simulink model "NonLin1C"  (R2019b)
settings: Solver=ode15s  StartTime=0.0  StopTime=200  FixedStep=0.1  RelTol=1e-3
values from neighbouring files (symbols this model uses):
  A_n = 0.05 * pi / 180    (= 0.000872664625997)    [Proj1C.m]
  g = 9.81    [Proj1C.m]
  K = 3    [Proj1C.m]
  L = 1    [Proj1C.m]
  M = 0.06    [Proj1C.m]
  omega_n = 200    [Proj1C.m]
  w_nonlin = W/8    (= 0.0109)    [Proj1C.m]
libraries: cstblocks x1
settings Model: NumberOfSteps=10  Creator=kmfrick  LastModifiedBy=kmfrick
settings SolverCC: ConcurrentTasks=on

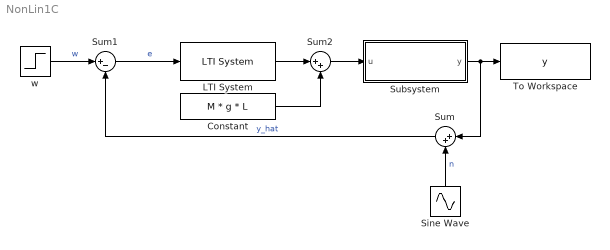
== system NonLin1C ==
  Constant : Constant  Value=M * g * L
  LTI System : cstblocks/LTI System  sys=R_opt  IC=[]
  Sine Wave : Sin  Amplitude=A_n  Frequency=omega_n  SampleTime=0
  Subsystem : Subsystem
  Sum : Sum  Inputs=|++
  Sum1 : Sum  Inputs=|+-
  Sum2 : Sum  Inputs=|++
  To Workspace : ToWorkspace  VariableName=y  SaveFormat=Timeseries  SampleTime=-1
  w : Step  Time=2  Before=pi/2  After=w_nonlin + pi/2  SampleTime=0
  wires:
  Sine Wave/1 -> Sum/2  "n"
  Sum/1 -> Sum1/2  "y_hat"
  Sum1/1 -> LTI System/1  "e"
  LTI System/1 -> Sum2/1
  Constant/1 -> Sum2/2
  w/1 -> Sum1/1  "w"
  Sum2/1 -> Subsystem/1(u)
  Subsystem/1(y) -> To Workspace/1, Sum/1

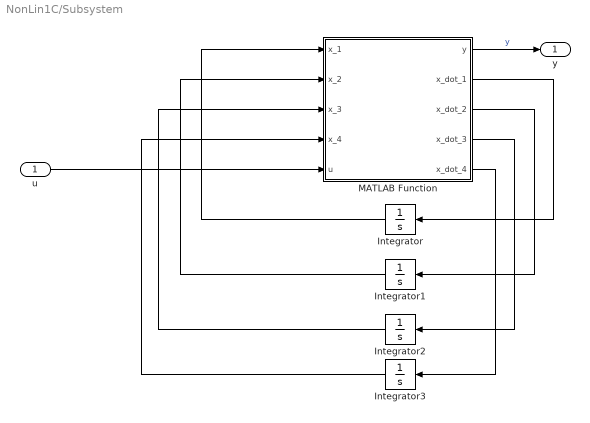
== system NonLin1C/Subsystem ==
  u : Inport
  Integrator : Integrator  InitialCondition=pi/2
  Integrator1 : Integrator
  Integrator2 : Integrator  InitialCondition=M *g * L / K + pi/2
  Integrator3 : Integrator
  MATLAB Function : MATLAB Function  TreatAsAtomicUnit=on
  y : Outport
  wires:
  Integrator1/1 -> MATLAB Function/2(x_2)
  MATLAB Function/3(x_dot_2) -> Integrator1/1
  MATLAB Function/5(x_dot_4) -> Integrator3/1
  Integrator/1 -> MATLAB Function/1(x_1)
  MATLAB Function/4(x_dot_3) -> Integrator2/1
  Integrator2/1 -> MATLAB Function/3(x_3)
  MATLAB Function/2(x_dot_1) -> Integrator/1
  Integrator3/1 -> MATLAB Function/4(x_4)
  u/1 -> MATLAB Function/5(u)
  MATLAB Function/1(y) -> y/1  "y"

== matlab function NonLin1C/Subsystem/MATLAB Function ==
  data: x_1 input size=1; x_2 input size=1; x_3 input size=1; x_4 input size=1; u input size=1; y output size=1; x_dot_1 output size=1; x_dot_2 output size=1; x_dot_3 output size=1; x_dot_4 output size=1
function [y, x_dot_1, x_dot_2, x_dot_3, x_dot_4] = NonLin1C(x_1, x_2, x_3, x_4, u)

omega_n = 200;
A_n = 0.05;
B_n = 20;
y_ref = pi/2;

%% Definizione dei parametri del sistema

g = 9.81;
K = 3;
ro = 0.2;
L = 1;
I = 0.01;
J = 0.02;
M = 0.06;


x_dot_1 = x_2;
x_dot_2 = (-M * g * L * sin (x_1) - K * (x_1 - x_3) - ro * (x_2 - x_4)) / J;
x_dot_3 = x_4;
x_dot_4 = (K * (x_1 - x_3) + ro * (x_2 - x_4) + u) / I;

y = x_1;

end
